simulink model "sixdof_v4"  (R2025b)
settings: Solver=ode45  StartTime=0.0  StopTime=300  FixedStep=1e-3  RelTol=1e-6  EnableMultiTasking=on
values from neighbouring files (symbols this model uses):
  antidive = 0.0    (= 0)    [init6dof_v4.m]
  antisquat = 0.0    (= 0)    [init6dof_v4.m]
  Bs = [1100 1100 1200 1200]    [init6dof_v4.m]
  c1s = [3  3  3  3]    [init6dof_v4.m]
  c2s = [7  7  7  7]    [init6dof_v4.m]
  Cfacs = [1.5  1.5  1.5  1.5]    [init6dof_v4.m]
  cruise = 1    [init6dof_v4.m]
  Cs = [1.4  1.4  1.4  1.4]    [init6dof_v4.m]
  dt = 0.1    [init6dof_v4.m]
  Es = [-0.2  -0.2  -0.2  -0.2]    [init6dof_v4.m]
  fdb = [0, 0, 0.5, 0.5]    [init6dof_v4.m]
  ftrack = 1.5    [init6dof_v4.m]
  hcg = 0.4    [init6dof_v4.m]
  hfrc = 0.1    [init6dof_v4.m]
  hrrc = 0.4    [init6dof_v4.m]
  I = [ixx, 0, -ixz; 0, iyy, 0; -ixz, 0, izz]    [init6dof_v4.m]
  Ic = 100    [init6dof_v4.m]
  invI = inv(I)    [init6dof_v4.m]
  Iw = [15 15 2 2]    [init6dof_v4.m]
  Karbf = stabf*180/pi    (= 0)    [init6dof_v4.m]
  Karbr = stabr*180/pi    (= 0)    [init6dof_v4.m]
  Kc = 500    [init6dof_v4.m]
  Kseff = 1./(1./Ks + 1./Kts)    [init6dof_v4.m]
  l = 2.83    [init6dof_v4.m]
  M = mf + mr    (= 1400)    [init6dof_v4.m]
  mu = 0.99*o4    [init6dof_v4.m]
  rc = [a, a, -b, -b ... (first row only)    [init6dof_v4.m]
  road = road * road_scale    [init6dof_v4.m]
  rr = 0.3    [init6dof_v4.m]
  rtrack = 1.5    [init6dof_v4.m]
  tau = 0.025    [init6dof_v4.m]
  tfby2 = ftrack/2    (= 0.75)    [init6dof_v4.m]
  TINY = 1e-5    (= 1e-05)    [init6dof_v4.m]
  trby2 = rtrack/2    (= 0.75)    [init6dof_v4.m]
  u0 = 5    [init6dof_v4.m]
  w0 = u0/rr*ones(4,1)    [init6dof_v4.m]
  woff = [wf; wf; wr; wr]/2    [init6dof_v4.m]
  x0 = zeros(10,1)    [init6dof_v4.m]
  Zrds = [16000  16000  16000  16000]    [init6dof_v4.m]
undefined symbols (not defined in the file or in its folder): cruise_params, steer_params
settings Model: Creator=ttmcb  LastModifiedBy=User
settings SolverCC: AlgebraicLoopSolver=TrustRegion
settings DataIOCC: SaveFormat=Array  SignalLoggingSaveFormat=ModelDataLogs  SaveOutput=off  SignalLogging=off  DSMLogging=off  ReturnWorkspaceOutputs=off  TimeSaveName=t
settings OptimizationCC: ExpressionDepthLimit=2147483647.0  InitFltsAndDblsToZero=on  LifeSpan=inf
settings DebuggingCC: AlgebraicLoopMsg=none  ArtificialAlgebraicLoopMsg=none  SaveWithParameterizedLinksMsg=none  UnderspecifiedInitializationDetection=Classic  MergeDetectMultiDrivingBlocksExec=none  SignalResolutionControl=TryResolveAllWithWarning  MultiTaskDSMMsg=warning  MultiTaskCondExecSysMsg=none  FcnCallInpInsideContextMsg=warning  UnconnectedInputMsg=warning  UnconnectedOutputMsg=warning  UnconnectedLineMsg=warning  StateNameClashWarn=warning  SFUnexpectedBacktrackingDiag=warning  SFNoUnconditionalDefaultTransitionDiag=warning  SFExecutionAtInitializationDiag=none  ArithmeticOperatorsInVariantConditions=warning
settings HardwareCC: ProdBitPerPointer=32.0  ProdBitPerSizeT=32.0  ProdBitPerPtrDiffT=32.0  ProdLargestAtomicFloat=None  ProdIntDivRoundTo=Undefined  ProdEndianess=Unspecified  ProdWordSize=32.0  ProdHWDeviceType=32-bit Generic  TargetHWDeviceType=32-bit Generic
settings ModelReferenceCC: PropagateSignalLabelsOutOfModel=off
settings SFSimCC: SimUseLocalCustomCode=off  SimParseCustomCode=off  CustomCodeUndefinedFunction=UseInterfaceOnly
settings RTWCC: GenCodeOnly=on  RTWUseLocalCustomCode=off  CustomInclude=c:\include  CustomSource=grt_shell.c  GPUComputeCapability=3.5
settings CodeAppCC: StateflowObjectComments=on
settings GRTTargetCC: TargetFcnLib=ansi_tfl_tmw.mat  TargetLangStandard=C89/C90 (ANSI)  CombineOutputUpdateFcns=off  GRTInterface=on
settings ConfigComp: CovMetricSettings=dw  CovSaveCumulativeToWorkspaceVar=on  CovSaveSingleToWorkspaceVar=on  CovExternalEMLEnable=off

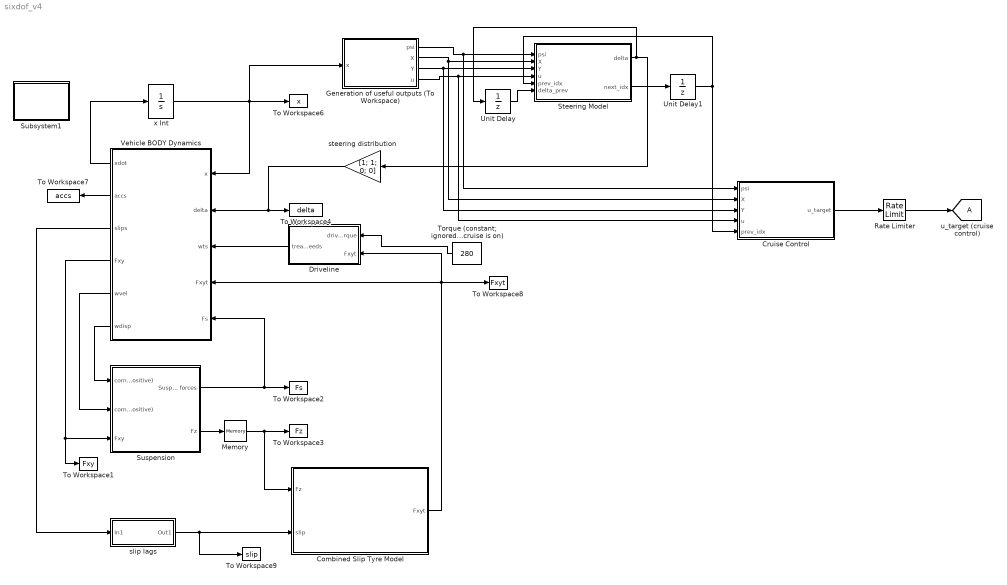
== system sixdof_v4 ==
  " Combined Slip Tyre Model" : MATLAB Function  TreatAsAtomicUnit=on
  " Vehicle BODY Dynamics" : MATLAB Function  TreatAsAtomicUnit=on
      settings: MinAlgLoopOccurrences=on
  Cruise Control : MATLAB Function  TreatAsAtomicUnit=on
  Driveline : Subsystem
      mask Display: disp('DRIVELINE')
  Generation of useful outputs (To Workspace) : Subsystem
  Memory : Memory  InitialCondition=woff
  Rate Limiter : RateLimiter  RisingSlewLimit=4  FallingSlewLimit=-4  SampleTimeMode=inherited
  Steering Model : MATLAB Function  TreatAsAtomicUnit=on
  Subsystem1 : Subsystem  Tag=BUIILD  Description=disp('BUILD')
      settings: OpenFcn=init6dof
      mask Display: disp('RUN\nInit6dof.m')
  Suspension : Subsystem
      mask Display: disp('SUSPENSION')
  To Workspace1 : ToWorkspace  VariableName=Fxy
  To Workspace2 : ToWorkspace  VariableName=Fs
  To Workspace3 : ToWorkspace  VariableName=Fz
  To Workspace4 : ToWorkspace  VariableName=delta
  To Workspace6 : ToWorkspace  VariableName=x
  To Workspace7 : ToWorkspace  VariableName=accs
  To Workspace8 : ToWorkspace  VariableName=Fxyt
  To Workspace9 : ToWorkspace  VariableName=slip
  Torque (constant; ignored if cruise is on) : Constant  Value=280
  Unit Delay : UnitDelay  SampleTime=dt  HasFrameUpgradeWarning=on
  Unit Delay1 : UnitDelay  InitialCondition=1  SampleTime=dt  HasFrameUpgradeWarning=on
  slip lags : Subsystem
      mask Display: disp('Relaxation\nlags');
  steering distribution : Gain  Gain=[1; 1; 0; 0]
  u_target (cruise control) : Goto  TagVisibility=global
  x Int : Integrator  InitialCondition=x0
  wires:
  " Combined Slip Tyre Model"/1(Fxyt) -> " Vehicle BODY Dynamics"/4(Fxyt), Driveline/2(Fxyt), To Workspace8/1
  Suspension/1(Suspension forces) -> To Workspace2/1, " Vehicle BODY Dynamics"/5(Fs)
  Suspension/2(Fz) -> Memory/1
  slip lags/1(Out1) -> " Combined Slip Tyre Model"/2(slip), To Workspace9/1
  " Vehicle BODY Dynamics"/6(wdisp) -> Suspension/1(corner verticall displacements (down positive))
  " Vehicle BODY Dynamics"/5(wvel) -> Suspension/2(corner vertical velocities (down positive))
  " Vehicle BODY Dynamics"/4(Fxy) -> Suspension/3(Fxy), To Workspace1/1
  " Vehicle BODY Dynamics"/3(slips) -> slip lags/1(In1)
  " Vehicle BODY Dynamics"/1(xdot) -> x Int/1
  x Int/1 -> " Vehicle BODY Dynamics"/1(x), To Workspace6/1, Generation of useful outputs (To Workspace)/1(x)
  " Vehicle BODY Dynamics"/2(accs) -> To Workspace7/1
  Torque (constant; ignored if cruise is on)/1 -> Driveline/1(drive or brake torque)
  Driveline/1(tread speeds) -> " Vehicle BODY Dynamics"/3(wts)
  steering distribution/1 -> " Vehicle BODY Dynamics"/2(delta), To Workspace4/1
  Memory/1 -> " Combined Slip Tyre Model"/1(Fz), To Workspace3/1
  Generation of useful outputs (To Workspace)/1(psi) -> Cruise Control/1(psi), Steering Model/1(psi)
  Generation of useful outputs (To Workspace)/2(X) -> Steering Model/2(X), Cruise Control/2(X)
  Generation of useful outputs (To Workspace)/3(Y) -> Steering Model/3(Y), Cruise Control/3(Y)
  Steering Model/1(delta) -> Unit Delay/1, steering distribution/1
  Unit Delay/1 -> Steering Model/6(delta_prev)
  Steering Model/2(next_idx) -> Unit Delay1/1
  Unit Delay1/1 -> Cruise Control/5(prev_idx), Steering Model/5(prev_idx)
  Generation of useful outputs (To Workspace)/4(u) -> Steering Model/4(u), Cruise Control/4(u)
  Cruise Control/1(u_target) -> Rate Limiter/1
  Rate Limiter/1 -> u_target (cruise control)/1

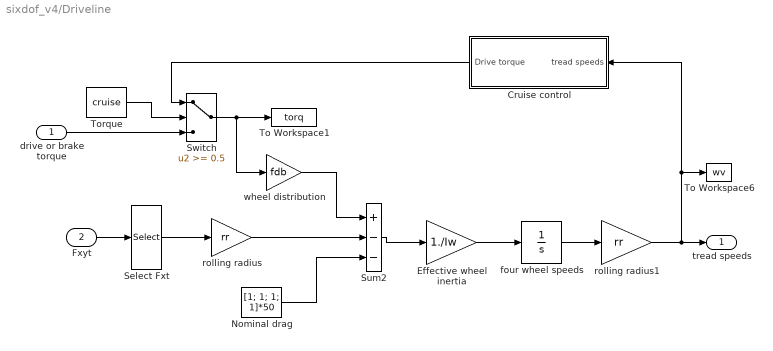
== system sixdof_v4/Driveline ==
  drive or brake torque : Inport
  Fxyt : Inport  Port=2
  Cruise control : Subsystem
  Effective wheel inertia : Gain  Gain=1./Iw
  Nominal drag : Constant  Value=[1; 1; 1; 1]*50
  "Select Fxt " : Selector  InputPortWidth=8  IndexOptions=Index vector (dialog)  Indices=[1:4]  OutputSizes=1
  Sum2 : Sum  Inputs=+--
  Switch : Switch  Threshold=0.5  SaturateOnIntegerOverflow=off  InputSameDT=off
  To Workspace1 : ToWorkspace  VariableName=torq
  To Workspace6 : ToWorkspace  VariableName=wv
  Torque : Constant  Value=cruise
  four wheel speeds : Integrator  InitialCondition=w0  LowerSaturationLimit=0
  rolling radius : Gain  Gain=rr
  rolling radius1 : Gain  Gain=rr
  wheel distribution : Gain  Gain=fdb
  tread speeds : Outport
  wires:
  rolling radius1/1 -> tread speeds/1, To Workspace6/1, Cruise control/1(tread speeds)
  Sum2/1 -> Effective wheel inertia/1
  four wheel speeds/1 -> rolling radius1/1
  "Select Fxt "/1 -> rolling radius/1
  Fxyt/1 -> "Select Fxt "/1
  Effective wheel inertia/1 -> four wheel speeds/1
  rolling radius/1 -> Sum2/2
  wheel distribution/1 -> Sum2/1
  Cruise control/1(Drive torque) -> Switch/1
  drive or brake torque/1 -> Switch/3
  Torque/1 -> Switch/2
  Switch/1 -> wheel distribution/1, To Workspace1/1
  Nominal drag/1 -> Sum2/3

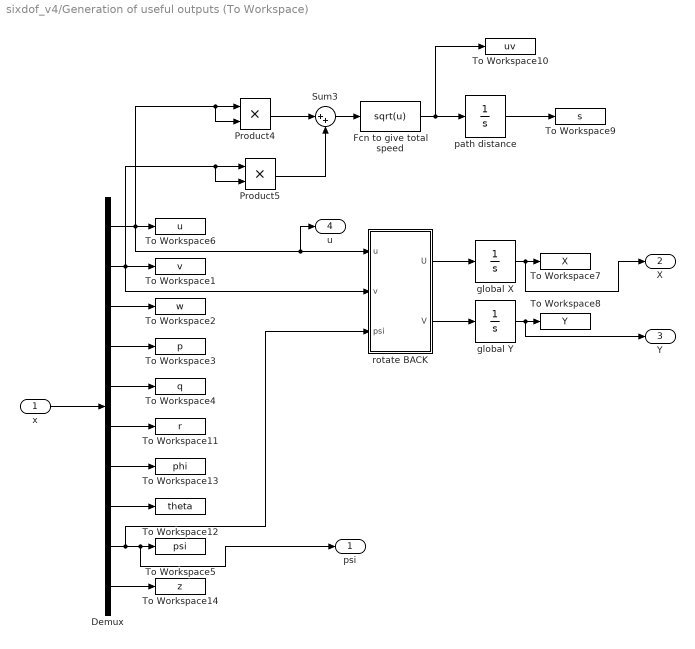
== system sixdof_v4/Generation of useful outputs (To Workspace) ==
  x : Inport
  Demux : Demux  Outputs=10
  Fcn to give total speed : Fcn  Expr=sqrt(u)
  Product4 : Product  RndMeth=Zero
  Product5 : Product  RndMeth=Zero
  Sum3 : Sum  Inputs=|++
  To Workspace1 : ToWorkspace  VariableName=v
  To Workspace10 : ToWorkspace  VariableName=uv
  To Workspace11 : ToWorkspace  VariableName=r
  To Workspace12 : ToWorkspace  VariableName=theta
  To Workspace13 : ToWorkspace  VariableName=phi
  To Workspace14 : ToWorkspace  VariableName=z
  To Workspace2 : ToWorkspace  VariableName=w
  To Workspace3 : ToWorkspace  VariableName=p
  To Workspace4 : ToWorkspace  VariableName=q
  To Workspace5 : ToWorkspace  VariableName=psi
  To Workspace6 : ToWorkspace  VariableName=u
  To Workspace7 : ToWorkspace  VariableName=X
  To Workspace8 : ToWorkspace  VariableName=Y
  To Workspace9 : ToWorkspace  VariableName=s
  global X : Integrator  LowerSaturationLimit=0
  global Y : Integrator  LowerSaturationLimit=0
  path distance : Integrator  LowerSaturationLimit=0
  rotate BACK : Subsystem
  psi : Outport
  X : Outport  Port=2
  Y : Outport  Port=3
  u : Outport  Port=4
  wires:
  Demux/1 -> To Workspace6/1, Product4/1, Product4/2, u/1, rotate BACK/1(u)
  Demux/2 -> To Workspace1/1, Product5/1, Product5/2, rotate BACK/2(v)
  Demux/3 -> To Workspace2/1
  Demux/4 -> To Workspace3/1
  Demux/5 -> To Workspace4/1
  x/1 -> Demux/1
  global X/1 -> X/1, To Workspace7/1
  global Y/1 -> Y/1, To Workspace8/1
  Product4/1 -> Sum3/1
  Product5/1 -> Sum3/2
  Sum3/1 -> Fcn to give total speed/1
  Fcn to give total speed/1 -> path distance/1, To Workspace10/1
  path distance/1 -> To Workspace9/1
  rotate BACK/1(U) -> global X/1
  rotate BACK/2(V) -> global Y/1
  Demux/6 -> To Workspace11/1
  Demux/7 -> To Workspace13/1
  Demux/8 -> To Workspace12/1
  Demux/9 -> psi/1, To Workspace5/1, rotate BACK/3(psi)
  Demux/10 -> To Workspace14/1

== system sixdof_v4/Subsystem1 ==

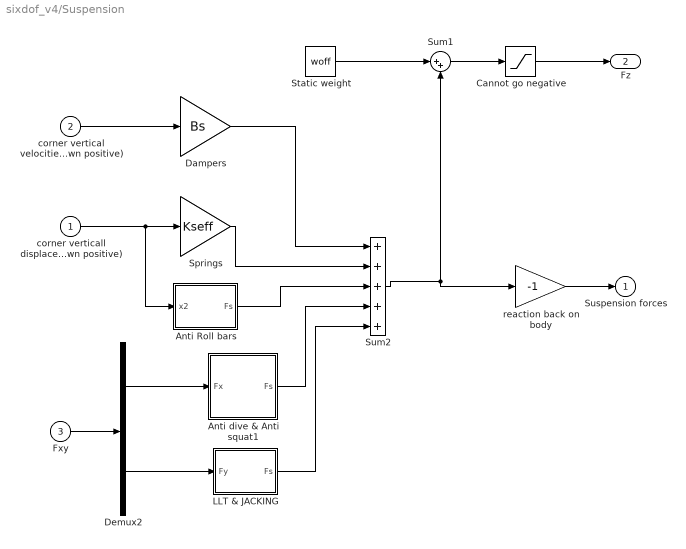
== system sixdof_v4/Suspension ==
  corner verticall displacements (down positive) : Inport
  corner vertical velocities (down positive) : Inport  Port=2
  Fxy : Inport  Port=3
  Anti Roll bars : Subsystem
  Anti dive & Anti squat1 : Subsystem
  Cannot go negative : Saturate  UpperLimit=inf  LowerLimit=TINY
  Dampers : Gain  Gain=Bs  SaturateOnIntegerOverflow=on  OutDataTypeStr=Inherit: Same as input  ParamDataTypeStr=Inherit: Same as input
  Demux2 : Demux  Outputs=[4,4]
  LLT & JACKING : Subsystem
  Springs : Gain  Gain=Kseff  SaturateOnIntegerOverflow=on  OutDataTypeStr=Inherit: Same as input  ParamDataTypeStr=Inherit: Same as input
  Static weight : Constant  Value=woff
  Sum1 : Sum  Inputs=|++
  Sum2 : Sum  Inputs=+++++  InputSameDT=on  SaturateOnIntegerOverflow=on  OutDataTypeStr=Inherit: Same as first input
  reaction back on body : Gain  Gain=-1  SaturateOnIntegerOverflow=on  OutDataTypeStr=Inherit: Same as input  ParamDataTypeStr=Inherit: Same as input
  Suspension forces : Outport
  Fz : Outport  Port=2
  wires:
  Cannot go negative/1 -> Fz/1
  corner vertical velocities (down positive)/1 -> Dampers/1
  corner verticall displacements (down positive)/1 -> Springs/1, Anti Roll bars/1(x2)
  Fxy/1 -> Demux2/1
  Demux2/1 -> Anti dive & Anti squat1/1(Fx)
  Demux2/2 -> LLT & JACKING/1(Fy)
  Dampers/1 -> Sum2/1
  Springs/1 -> Sum2/2
  reaction back on body/1 -> Suspension forces/1
  Sum1/1 -> Cannot go negative/1
  Sum2/1 -> reaction back on body/1, Sum1/2
  Static weight/1 -> Sum1/1
  LLT & JACKING/1(Fs) -> Sum2/5
  Anti dive & Anti squat1/1(Fs) -> Sum2/4
  Anti Roll bars/1(Fs) -> Sum2/3

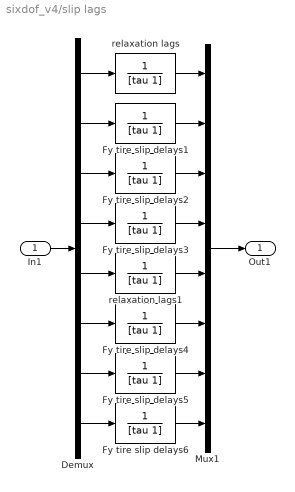
== system sixdof_v4/slip lags ==
  In1 : Inport
  Demux : Demux  Outputs=8
  Fy tire slip delays{1..6} (6 alike) : TransferFcn  Numerator=1  Denominator=[tau 1]
  Mux1 : Mux  Inputs=8
  relaxation lags : TransferFcn  Numerator=1  Denominator=[tau 1]
  relaxation lags1 : TransferFcn  Numerator=1  Denominator=[tau 1]
  Out1 : Outport
  wires:
  Mux1/1 -> Out1/1
  In1/1 -> Demux/1
  Demux/4 -> Fy tire slip delays3/1
  Demux/3 -> Fy tire slip delays2/1
  Demux/2 -> Fy tire slip delays1/1
  Demux/1 -> relaxation lags/1
  Fy tire slip delays3/1 -> Mux1/4
  Fy tire slip delays2/1 -> Mux1/3
  Fy tire slip delays1/1 -> Mux1/2
  relaxation lags/1 -> Mux1/1
  Demux/5 -> relaxation lags1/1
  Demux/6 -> Fy tire slip delays4/1
  Demux/7 -> Fy tire slip delays5/1
  Demux/8 -> Fy tire slip delays6/1
  relaxation lags1/1 -> Mux1/5
  Fy tire slip delays4/1 -> Mux1/6
  Fy tire slip delays5/1 -> Mux1/7
  Fy tire slip delays6/1 -> Mux1/8

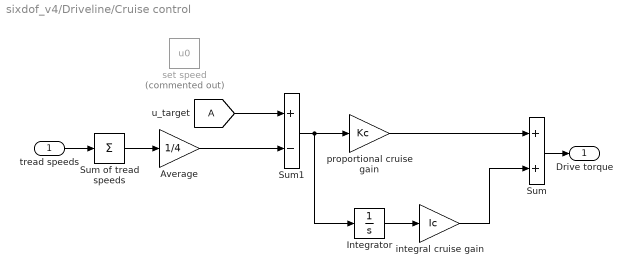
== system sixdof_v4/Driveline/Cruise control ==
  tread speeds : Inport
  Average : Gain  Gain=1/4
  Integrator : Integrator
  Sum : Sum
  Sum of tread speeds : Sum  Inputs=+
  Sum1 : Sum  Inputs=+-
  integral cruise gain : Gain  Gain=Ic
  proportional cruise gain : Gain  Gain=Kc
  set speed : Constant  Commented=on  Value=u0
  u_target : From  TagVisibility=global
  Drive torque : Outport
  wires:
  proportional cruise gain/1 -> Sum/1
  integral cruise gain/1 -> Sum/2
  Integrator/1 -> integral cruise gain/1
  Sum1/1 -> Integrator/1, proportional cruise gain/1
  Sum/1 -> Drive torque/1
  tread speeds/1 -> Sum of tread speeds/1
  Sum of tread speeds/1 -> Average/1
  Average/1 -> Sum1/2
  u_target/1 -> Sum1/1

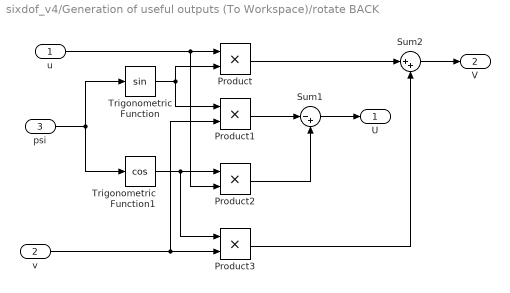
== system sixdof_v4/Generation of useful outputs (To Workspace)/rotate BACK ==
  u : Inport
  v : Inport  Port=2
  psi : Inport  Port=3
  Product{,1..3} (4 alike) : Product  RndMeth=Zero
  Sum1 : Sum  Inputs=|-+
  Sum2 : Sum  Inputs=|++
  Trigonometric Function : Trigonometry
  Trigonometric Function1 : Trigonometry  Operator=cos
  U : Outport
  V : Outport  Port=2
  wires:
  Trigonometric Function/1 -> Product/2, Product1/1
  Trigonometric Function1/1 -> Product2/1, Product3/1
  Product1/1 -> Sum1/1
  Product2/1 -> Sum1/2
  Sum1/1 -> U/1
  Product/1 -> Sum2/1
  Product3/1 -> Sum2/2
  Sum2/1 -> V/1
  psi/1 -> Trigonometric Function/1, Trigonometric Function1/1
  u/1 -> Product/1, Product2/2
  v/1 -> Product3/2, Product1/2

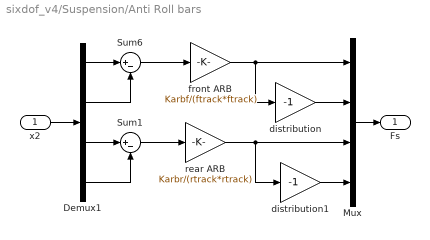
== system sixdof_v4/Suspension/Anti Roll bars ==
  x2 : Inport
  Demux1 : Demux
  Mux : Mux
  Sum1 : Sum  Inputs=|+-
  Sum6 : Sum  Inputs=|+-
  distribution : Gain  Gain=-1
  distribution1 : Gain  Gain=-1
  front ARB : Gain  Gain=Karbf/(ftrack*ftrack)
  rear ARB : Gain  Gain=Karbr/(rtrack*rtrack)
  Fs : Outport
  wires:
  Demux1/1 -> Sum6/1
  Demux1/2 -> Sum6/2
  Demux1/3 -> Sum1/1
  Demux1/4 -> Sum1/2
  Sum6/1 -> front ARB/1
  Sum1/1 -> rear ARB/1
  x2/1 -> Demux1/1
  Mux/1 -> Fs/1
  distribution1/1 -> Mux/4
  rear ARB/1 -> distribution1/1, Mux/3
  distribution/1 -> Mux/2
  front ARB/1 -> distribution/1, Mux/1

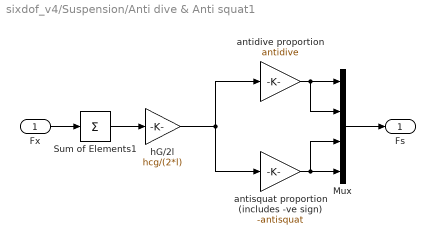
== system sixdof_v4/Suspension/Anti dive & Anti squat1 ==
  Fx : Inport
  Mux : Mux
  Sum of Elements1 : Sum  Inputs=+
  antidive proportion : Gain  Gain=antidive
  antisquat proportion (includes -ve sign) : Gain  Gain=-antisquat
  hG/2l : Gain  Gain=hcg/(2*l)
  Fs : Outport
  wires:
  hG/2l/1 -> antidive proportion/1, antisquat proportion (includes -ve sign)/1
  antisquat proportion (includes -ve sign)/1 -> Mux/3, Mux/4
  Fx/1 -> Sum of Elements1/1
  Mux/1 -> Fs/1
  antidive proportion/1 -> Mux/2, Mux/1
  Sum of Elements1/1 -> hG/2l/1

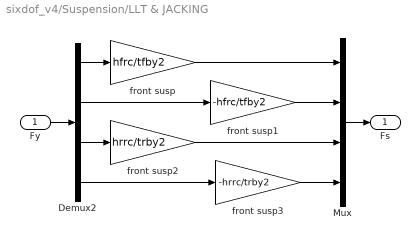
== system sixdof_v4/Suspension/LLT & JACKING ==
  Fy : Inport
  Demux2 : Demux
  Mux : Mux
  front susp : Gain  Gain=hfrc/tfby2
  front susp1 : Gain  Gain=-hfrc/tfby2
  front susp2 : Gain  Gain=hrrc/trby2
  front susp3 : Gain  Gain=-hrrc/trby2
  Fs : Outport
  wires:
  front susp/1 -> Mux/1
  Demux2/1 -> front susp/1
  front susp1/1 -> Mux/2
  Demux2/2 -> front susp1/1
  front susp2/1 -> Mux/3
  Demux2/3 -> front susp2/1
  front susp3/1 -> Mux/4
  Demux2/4 -> front susp3/1
  Fy/1 -> Demux2/1
  Mux/1 -> Fs/1

== matlab function sixdof_v4/Cruise Control ==
  settings: updateMethod=DISCRETE  sampleTime=dt
  data: psi input; X input; Y input; u input; u_target output; cruise_params parameter; prev_idx input; road parameter
function u_target = Cruise_control(psi, X, Y, u, cruise_params, prev_idx, road)
% CRUISE_CONTROL  Target speed based on look-ahead curvature.
%
%   Structurally identical to the Steering MATLAB Function block:
%     - Same sliding-window position search (Part 1)
%     - Same forward walk to build lookahead window (Part 2)
%   Then differs in what it does with the preview:
%     - Scans every A-B-C triplet inside the window for curvature (Part 3)
%     - Outputs  u_target = sqrt(ay_max * R_min)             (Part 4)
%
%   INPUTS
%     psi           – yaw angle [rad]  (port compatibility only)
%     X, Y          – vehicle CG position [m]
%     u             – current speed [m/s]
%     cruise_params – struct: .Tp, .ay_max (default 7.5), .u_min (default 2)
%     prev_idx      – shared index fed from the Steering next_idx output
%     road          – Nx2 [X Y] centreline [m]
%
%   OUTPUT
%     u_target      – target speed [m/s]  →  "set speed" in Simulink




    % ---- Parameters ----
    Tp     = cruise_params.Tp;
    ay_max = cruise_params.ay_max;
    u_min  = cruise_params.u_min;
    u_max  = cruise_params.u_max;
    % ---------------------------------------------------------------- %
    %  1. Find current segment – identical to Steering MLFB              %
    % ---------------------------------------------------------------- %
    search_window = 100;
    N = size(road, 1);

    idx      = prev_idx;
    min_dist = inf;

    start_k = prev_idx;
    end_k   = min(prev_idx + search_window, N - 1);

    % End simulation after reaching the end of the track
    for i = start_k : end_k
        p1 = road(i,   :);
        p2 = road(i+1, :);

        t_vec   = p2 - p1;
        seg_len = norm(t_vec);
        if seg_len < 1e-6, continue; end
        t_hat = t_vec / seg_len;

        v_vec    = [X, Y] - p1;
        proj_len = dot(v_vec, t_hat);

        % Calculate distance to segment
        curr_d = norm(v_vec - proj_len * t_hat);

        % Add penalty if outside segment to favour the correct segment
        if proj_len < 0 || proj_len > seg_len
            curr_d = curr_d + 10.0;
        end

        if curr_d < min_dist
            min_dist = curr_d;
            idx      = i;
        end
    end

    next_idx = idx;   % current best segment

    % ---------------------------------------------------------------- %
    %  2. Walk forward – identical to Steering MLFB (previewDist)       %
    % ---------------------------------------------------------------- %
    previewDist = max(5.0, u * Tp);   % same formula as steering

    travelled = 0;
    j = next_idx;
    while j < N - 1 && travelled < previewDist
        ds        = norm(road(j+1,:) - road(j,:));
        travelled = travelled + ds;
        j         = j + 1;
    end
    % j is now the far end of the lookahead window

    % ---------------------------------------------------------------- %
    %  3. Curvature scan – every A-B-C triplet in the window            %
    % ---------------------------------------------------------------- %
    R_min = inf;
    k     = next_idx;

    while k <= j - 2
        A = road(k,   :);
        B = road(k+1, :);
        C = road(k+2, :);

        r1     = B - A;
        r2     = C - B;
        mag_r1 = norm(r1);
        mag_r2 = norm(r2);

        if mag_r1 < 1e-6 || mag_r2 < 1e-6
            k = k + 1;
            continue;
        end

        delta_S     = (mag_r1 + mag_r2) / 2.0;
        cp_z        = r1(1)*r2(2) - r1(2)*r2(1);
        sin_dtheta  = max(-1.0, min(1.0, cp_z / (mag_r1 * mag_r2)));
        delta_theta = asin(sin_dtheta);
        kappa       = abs(delta_theta) / delta_S;

        if kappa > 1e-9
            R_local = 1.0 / kappa;
            if R_local < R_min
                R_min = R_local;
            end
        end

        k = k + 1;
    end

    % Straight ahead → treat as very large radius (free acceleration)
    if isinf(R_min)
        R_min = (u_max^2) / ay_max;
    end

    % ---------------------------------------------------------------- %
    %  4. Target speed  (v = sqrt(ay_max * R_min))                     %
    % ---------------------------------------------------------------- %
    u_target = sqrt(ay_max * R_min);
    u_target = max(u_target, u_min);
    u_target = min(u_target, u_max);
end

== matlab function sixdof_v4/Steering Model ==
  settings: updateMethod=DISCRETE  sampleTime=dt
  data: psi input; X input; Y input; u input; delta output; steer_params parameter; prev_idx input; delta_prev input; next_idx output; road parameter
function [delta, next_idx] = fcn(psi, X, Y, u, steer_params, prev_idx, delta_prev, road)


    % Extract Parameters
    Tp   = steer_params.Tp;
    Klat = steer_params.Klat;
    L    = steer_params.L;
    Kug  = steer_params.Kug;

    
    % Find Current Position S_G on Track
    % Search window from previous index
    search_window = 100; 
    N = size(road, 1);
    
    idx = prev_idx;
    min_dist = inf;
    
    start_k = prev_idx;
    end_k = min(prev_idx + search_window, N-1);
    
    % End simulation after reaching the end of the track
    
    for i = start_k : end_k
        p1 = road(i, :);
        p2 = road(i+1, :);
        
        t_vec = p2 - p1;
        seg_len = norm(t_vec);
        if seg_len < 1e-6, continue; end
        t_hat = t_vec / seg_len;
        
        v_vec = [X, Y] - p1;
        proj_len = dot(v_vec, t_hat);
        
        % Calculate distance to segment
        curr_d = norm(v_vec - proj_len * t_hat);
        
        % Add penalty if outside segment to favor the road segment
        if proj_len < 0 || proj_len > seg_len
            curr_d = curr_d + 10.0; 
        end
        
        if curr_d < min_dist
             min_dist = curr_d;
             idx = i;
        end
    end
    
    next_idx = idx; 
    
    % Calculate Kinematic Preview Point P 
    % Standard Steady State Radius R (Eq 2)
    if abs(delta_prev) < 1e-5
        R = inf;
    else
        R = (L + Kug * u^2) / delta_prev;
    end
    
    % Heading/Normal vectors
    tG = [cos(psi), sin(psi)];
    nG = [-sin(psi), cos(psi)]; % Normal to Left
    
    if isinf(R)
        % Straight line projection
        P = [X, Y] + u * Tp * tG;
    else
        % Circular projection (Eq 5)
        % Center of curvature O = G + R * nG
        O = [X, Y] + R * nG;
        
        % Angle traversed theta (Eq 4)
        theta = (u * Tp) / R;
        
        % Vector from O to G is -R*nG. Rotate it by theta.
        v = -R * nG;
        
        cos_t = cos(theta);
        sin_t = sin(theta);
        
        % 2D Rotation
        v_rot = [v(1)*cos_t - v(2)*sin_t, v(1)*sin_t + v(2)*cos_t];
        
        P = O + v_rot;
    end
    
    % Lateral Error Calculation
    % Find segment P falls on.
    % Search forward from 'next_idx' since P is ahead.
    
    best_d = inf;
    best_idx = next_idx;
    found_valid = false;
    
    search_fwd = 200; % Larger window for lookahead
    
    for k = next_idx : min(next_idx + search_fwd, N-1)
        curr_S = road(k, :);
        next_S = road(k+1, :);
        
        seg_vec = next_S - curr_S;
        s_len = norm(seg_vec);
        if s_len < 1e-6, continue; end
        t_hat_L = seg_vec / s_len;
        
        p_vec = P - curr_S;
        proj = dot(p_vec, t_hat_L);
        
        % Check if valid segment (Eq 9)
        if proj >= -1.0 && proj <= s_len + 1.0 % Allow 1m slack
             % Valid segment
             n_L_local = [-t_hat_L(2), t_hat_L(1)]; % Left Normal
             dist = dot(p_vec, n_L_local);
             
             % Find smallest valid d (closest segment involved)
             if abs(dist) < abs(best_d)
                 best_d = dist;
                 found_valid = true;
             end
        end
    end
    
    if ~found_valid             
        % Projection onto the 'next_idx' tangent extended.
        curr_S = road(next_idx, :);
        next_S = road(next_idx+1, :);
        seg_vec = next_S - curr_S;
        t_hat_L = seg_vec / norm(seg_vec);
        n_L_local = [-t_hat_L(2), t_hat_L(1)];
        best_d = dot(P - curr_S, n_L_local);
    end
    
    d_lat = best_d;
    
    %Steering Update (Eq 11) 
    % delta(k+1) = delta(k) - Klat * d
    delta_cmd = delta_prev - Klat * d_lat;
    
    % Saturation
    delta_max = deg2rad(35);
    delta = max(-delta_max, min(delta_cmd, delta_max));
    
end

== matlab function sixdof_v4/ Vehicle BODY Dynamics ==
  data: x input; delta input; wts input; Fxyt input; Fs input; M parameter; invI parameter; I parameter; rc parameter; hcg parameter; xdot output; accs output; slips output; Fxy output; wvel output; wdisp output
function [xdot,accs,slips,Fxy,wvel,wdisp] = BODY(x,delta,wts,Fxyt,Fs,M,invI,I,rc,hcg)
%
% Embedded Matlab function to calculate vehicle body
% accelerations (state derivatives).
%

% Fixed parameters :
o4 = ones(1,4);
TINY = 1e-5;
TINYrow = TINY*o4;

% Variables renamed from states :
V = x(1:3);
w = x(4:6);
theta = x(7:9);
z = x(10);

%%%%%%%%%%%%%%%%%%%%%%%%%%%%%%%%%%%%%%%%%%%%%%%%%%%%
% Calculate velocities at tyre contact patches, in 
% Tyre axis system :

cornervels = V*o4 + cross(w*o4,rc);
wvel = cornervels(3,:)';

uvel = cornervels(1,:)';
vvel = cornervels(2,:)';

cornerdisp_rot = cross(theta*o4,rc);
wdisp = z*o4' + cornerdisp_rot(3,:)';

cosdels = cos(delta);
sindels = sin(delta);

% Rotate into tyre axis system :
uts = cosdels.*uvel + sindels.*vvel;
vts = cosdels.*vvel - sindels.*uvel;


%%%%%%%%%%%%%%%%%%%%%%%%%%%%%%%%%%%%%%%%%%%%%%%%%%%%
% Lateral and longitudinal slip :
udens = max([abs(uts');TINYrow])';
sys = -vts ./ udens;
sxs = (wts - uts) ./ udens;
slips = [sxs; sys];
    

%%%%%%%%%%%%%%%%%%%%%%%%%%%%%%%%%%%%%%%%%%%%%%%%%%%%
% Calculate tyre forces in body axis system
Fxt = Fxyt(1:4);
Fyt = Fxyt(5:8);

Fx = cosdels.*Fxt - sindels.*Fyt;
Fy = cosdels.*Fyt + sindels.*Fxt;
Fxy = [Fx; Fy];

%%%%%%%%%%%%%%%%%%%%%%%%%%
% Vehicle BODY dynamics :
% Position of tyre contact patches wrt CG :
rs = rc;
rs(3,:) = rs(3,:) - wdisp' + hcg;

% Forces :
F = [Fxy(1:4), Fxy(5:8), Fs];
sumF = sum(F)';

% Moments :
rxF = cross(rs',F);
Mom = sum(rxF)';

% Derivatives :
acctran = sumF/M;
Vdot = acctran - cross(w,V);

accrot = invI*Mom;
wdot = invI*(Mom - cross(w,I*w));

xdot = [Vdot; wdot; w; V(3)];
accs = [acctran; accrot];

return;

== matlab function sixdof_v4/ Combined Slip Tyre Model ==
  data: Fz input size=4; Fxyt output size=8; slip input; c1s parameter; c2s parameter; Zrds parameter; Cfacs parameter; Cs parameter; Es parameter; mu parameter
function Fxyt  = TYRES(Fz,slip,c1s,c2s,Zrds,Cfacs,Cs,Es,mu)
%
% Embedded Matlab function to calculate combined slip
% tyre model, using basic Pacejka model, and functions
% for peak load and cornering / long stiffness.
% In this version, all four tyres are calcalated concurrently
% so all variables and parameters are 4x1 vectors.
%
% Cornering stiffness and mu variations with load nominally follow 
% guidelines in 'Tires, Suspension and Handling' by John Dixon.
%

Fxyt = zeros(8,1);

% Loop necessary to avoid division by zero in calcs, and because embedded Matlab is limited (no ./).
for i=1:4,
    % Identify all variables and parameters within the loop :
    c1 = c1s(i);
    c2 = c2s(i);
    Zrd = Zrds(i);
    Cfac = Cfacs(i);
    C = Cs(i);
    E = Es(i);

    sx = slip(i);
    sy = slip(i+4);
    Zt = Fz(i);
    
    % Cornering stiffnesses :
    Ca = c1*Zrd*(1-exp(-c2*Zt/Zrd));
    Cx = Ca*Cfac;

    % Peak forces :
    murat = (4*Zt/Zrd)^(-0.15);     % 4*Zt same as Zrd/4 (per tyre rating here)
    murat = min([1.6, murat]);
    Fyp = mu(i)*murat*Zt;
    Fxp = Fyp;

    % Step 1, Total slip :
    sxbar = Cx*sx/Fxp;
    sybar = Ca*sy/Fyp;
    sr = sqrt(sxbar^2 + sybar^2);

    % Step 2, Magic formula :
    Fr = sin( C*atan(sr/C - E*(sr/C - atan(sr/C))) );

    % Step3, eta0
    eta0 = Ca*Fxp / (Cx*Fyp);
    
    % Step4,
    % Calulate eta(sr) (interpolation function)
    if sr < (2*pi),
        eta = 0.5*(1+eta0) - 0.5*(1-eta0)*cos(0.5*sr);
    else
        eta = 1;
    end;
    if sxbar~=0,   % This logic needed to avoid division by zero in Eq 1
        % Equation 1 :
        rho = eta*sybar/(eta0*sxbar);
        % Equation 2 :
        % In this last equation, sign(sx) is used, since the sign of rho will then determine sign(Fy) correctly.
        Fxbar = sign(sx)*Fr/sqrt(1 + rho*rho);
        Fybar = Fxbar*rho;
    else,       % sxbar is identically zero, Fr goes to Fy
        Fxbar = 0;
        Fybar = sign(sy)*Fr;
    end;

    % Step 5 :
    Fxyt(i) = Fxbar*Fxp;
    Fxyt(i+4) = Fybar*Fyp;
    
end;


return;
